simulink model "VisionVehicleDetector"  (R2022b)
settings: Solver=FixedStepAuto  StartTime=0.0  StopTime=scenario.StopTime  RelTol=1e-3  EnableMultiTasking=on
settings Model: Creator=The MathWorks, Inc.  LastModifiedBy=Administrator
settings SolverCC: AlgebraicLoopSolver=TrustRegion  MaxZcPerStep=1
settings DataIOCC: SaveOutput=off  SaveTime=off  ReturnWorkspaceOutputs=off
settings OptimizationCC: DefaultParameterBehavior=Inlined  InlineInvariantSignals=on  EnhancedBackFolding=on  PassReuseOutputArgsAs=Individual arguments  ZeroExternalMemoryAtStartup=off  ZeroInternalMemoryAtStartup=off  InitFltsAndDblsToZero=on  EfficientFloat2IntCast=on  OptimizeBlockOrder=speed  DifferentSizesBufferReuse=on  OptimizationCustomize=off  EfficientTunableParamExpr=on
settings DebuggingCC: ParameterPrecisionLossMsg=none  ParameterTunabilityLossMsg=error  UnconnectedInputMsg=warning  UnconnectedOutputMsg=warning  UnconnectedLineMsg=warning  PregeneratedLibrarySubsystemCodeDiagnostic=none  SFMachineParentedDataDiag=warning  ArithmeticOperatorsInVariantConditions=warning
settings HardwareCC: ProdLongLongMode=on  TargetLongLongMode=on
settings ModelReferenceCC: EnableRefExpFcnMdlSchedulingChecks=on  PropagateVarSize=During execution
settings SFSimCC: SimUseLocalCustomCode=off  SimTargetLang=C++
settings RTWCC: Description=Embedded Coder  SystemTargetFile=ert.tlc  TemplateMakefile=ert_default_tmf  RTWVerbose=off  RTWUseLocalCustomCode=off  BuildConfiguration=Faster Runs  CodeExecutionProfiling=on  CodeProfilingSaveOptions=AllData  TargetLang=C++  GenerateGPUCode=CUDA  DLTargetLibrary=cudnn  DLArmComputeVersion=19.05
settings CodeAppCC: ForceParamTrailComments=on  IgnoreCustomStorageClasses=off  OperatorAnnotations=on  SimulinkDataObjDesc=on  SFDataObjDesc=on  CustomSymbolStrGlobalVar=$N$M  CustomSymbolStrType=$N$M_T  CustomSymbolStrFcn=APV_$N$M$F  CustomSymbolStrMacro=$N$M  InsertBlockDesc=on
settings ERTTargetCC: TargetLangStandard=C++03 (ISO)  GenerateSampleERTMain=on  CombineSignalStateStructs=on  CodeInterfacePackaging=C++ class  SupportVariableSizeSignals=on  InlinedParameterPlacement=NonHierarchical  RootIOFormat=Structure reference  ERTCustomFileTemplate=example_file_process.tlc
settings ConfigComp: CovScope=ReferencedModels  CovIncludeTopModel=off

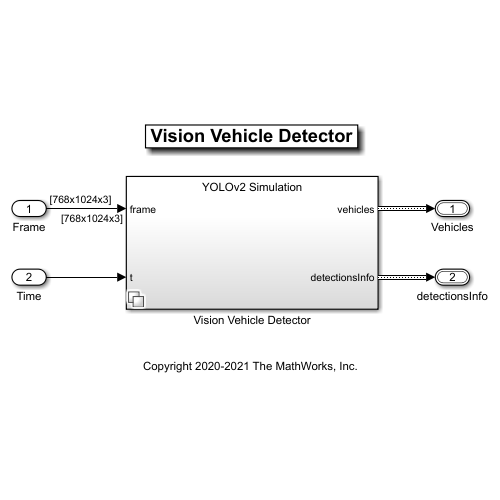
[thumbnail: Simulink's stored preview of the top-level diagram]
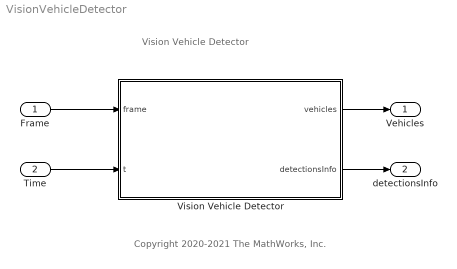
== system VisionVehicleDetector ==
  note: Copyright 2020-2021 The MathWorks, Inc.
  note: Vision Vehicle Detector
  Frame : Inport  OutDataTypeStr=uint8  PortDimensions=[768 1024 3]  SampleTime=[0.10000000000000001,0]
  Time : Inport  Port=2  OutDataTypeStr=double  PortDimensions=1  SampleTime=[0.10000000000000001,0]
  Vision Vehicle Detector : Subsystem  Variant=on  VariantControl=Choice
  Vehicles : Outport  OutDataTypeStr=Bus: BusVision  PortDimensions=[1 1]  SampleTime=[0.10000000000000001,0]  BusOutputAsStruct=on
  detectionsInfo : Outport  Port=2  OutDataTypeStr=Bus: BusVisionInfo  BusOutputAsStruct=on
  wires:
  Time/1 -> Vision Vehicle Detector/2(t)
  Frame/1 -> Vision Vehicle Detector/1(frame)
  Vision Vehicle Detector/1(vehicles) -> Vehicles/1
  Vision Vehicle Detector/2(detectionsInfo) -> detectionsInfo/1

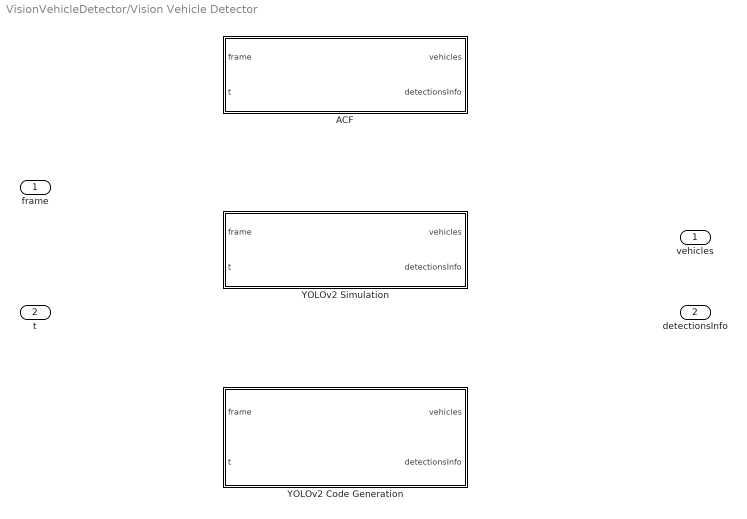
== system VisionVehicleDetector/Vision Vehicle Detector ==
  frame : Inport
  t : Inport  Port=2
  ACF : Subsystem  VariantControl="detectorVariant == \"ACF\""
  YOLOv2 Code Generation : MATLAB Function  TreatAsAtomicUnit=on  VariantControl="detectorVariant == \"YOLOv2 Code Generation\""
  YOLOv2 Simulation : Subsystem  VariantControl="detectorVariant == \"YOLOv2 Simulation\""
  vehicles : Outport  OutDataTypeStr=Bus: BusVision
  detectionsInfo : Outport  Port=2  OutDataTypeStr=Bus: BusVisionInfo

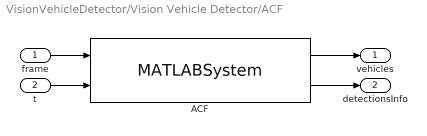
== system VisionVehicleDetector/Vision Vehicle Detector/ACF ==
  frame : Inport
  t : Inport  Port=2
  ACF : MATLABSystem  System=HelperVisionVehicleDetector  EnableDisplay=on  Detector=VehicleDetector.ACF  Camera=camera  SimulateUsing=Interpreted execution
      mask Type: HelperVisionVehicleDetector
      mask Display:
      | disp('HelperVisionVehicleDetector');
      | port_label('input',1,'frame');
      | port_label('input',2,'t');
      | port_label('output',1,'vehicles');
      | port_label('output',2,'detectionsInfo');
  vehicles : Outport
  detectionsInfo : Outport  Port=2  OutDataTypeStr=Bus: BusVisionInfo
  wires:
  frame/1 -> ACF/1
  t/1 -> ACF/2
  ACF/1 -> vehicles/1
  ACF/2 -> detectionsInfo/1

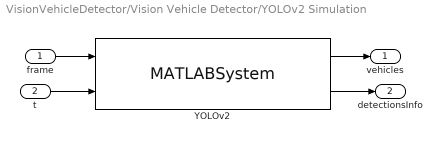
== system VisionVehicleDetector/Vision Vehicle Detector/YOLOv2 Simulation ==
  frame : Inport
  t : Inport  Port=2
  YOLOv2 : MATLABSystem  System=HelperVisionVehicleDetector  EnableDisplay=off  Detector=VehicleDetector.YOLOv2  Camera=camera  SimulateUsing=Interpreted execution
      mask Type: HelperVisionVehicleDetector
      mask Display:
      | disp('HelperVisionVehicleDetector');
      | port_label('input',1,'frame');
      | port_label('input',2,'t');
      | port_label('output',1,'vehicles');
      | port_label('output',2,'detectionsInfo');
  vehicles : Outport
  detectionsInfo : Outport  Port=2  OutDataTypeStr=Bus: BusVisionInfo
  wires:
  frame/1 -> YOLOv2/1
  t/1 -> YOLOv2/2
  YOLOv2/1 -> vehicles/1
  YOLOv2/2 -> detectionsInfo/1

== matlab function VisionVehicleDetector/Vision Vehicle Detector/YOLOv2 Code Generation ==
  settings: updateMethod=DISCRETE
  data: frame input; vehicles output Bus: BusVision; t input; detectionsInfo output Bus: BusVisionInfo
function [vehicles, detectionsInfo] = YOLOv2CodeGenWrapper(frame, t)

persistent vehicleDetector;
if(isempty(vehicleDetector))
    vehicleDetector = HelperVisionVehicleDetector('Detector', VehicleDetector.YOLOv2);
end
[vehicles, detectionsInfo] = step(vehicleDetector, frame, t);

end
